simulink model "threeStateSM_functionCallGenerator"  (R2024b)
settings: Solver=VariableStepAuto  StartTime=0.0  StopTime=10.0  RelTol=1e-3
libraries: simulink x1
settings Model: Creator=optimus  LastModifiedBy=optimus

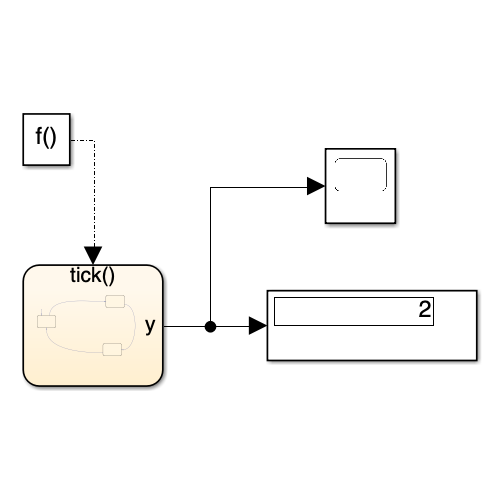
[thumbnail: Simulink's stored preview of the top-level diagram]
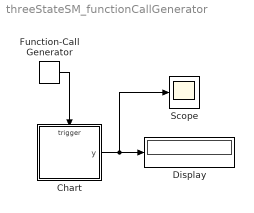
== system threeStateSM_functionCallGenerator ==
  Chart : Stateflow chart  TreatAsAtomicUnit=on
  Display : Display
  Function-Call Generator : simulink/Ports & Subsystems/Function-Call Generator  sample_time=1  numberOfIterations=1  DisallowWideOutput=off
  Scope : Scope
  wires:
  Chart/1(y) -> Scope/1, Display/1
  Function-Call Generator/1 -> Chart/Trigger

== stateflow chart threeStateSM_functionCallGenerator/Chart ==
  settings: executeAtInitialization=1
  state B
  state A
  state C
  A -> B : tick{y=1}
  B -> C : tick{y=2}
  (default) -> A
  C -> A : tick{y=3}
  data: y output
  events: tick input FUNCTION_CALL_EVENT
